simulink model "untitled"  (R2021a)
settings: Solver=VariableStepAuto  StartTime=0.0  StopTime=5  RelTol=1e-3
undefined symbols (not defined in the file or in its folder): sigbuilder_block
libraries: fuzblock x3
(part 2 of 4)

== matlab function untitled/MATLAB Function4 ==
  data: q input; C output; qd input
% Copyright (C) 2022 All rights reserved.
% Authors:     Seonghyeon Jo <cpsc.seonghyeon@gmail.com>
%
% Date:        Jan, 18, 2022
% 
% -------------------------------------------------
% Sawyer Robot 4-DoF
% get a coriolis matrix.
% -------------------------------------------------
% Equation)
%       c(q, dq)
%
% Input)
%       x   : Joint Position
%       dx  : Joint Velocity
% Output)
%       C  : Coriolis Matrix
%
% the following code has been tested on Matlab 2021a
function C = compute_C_4DOF(q,qd)
g=9.81
m1=1;m2=0.7;m3=0.35;
m12=m1+m2;
m23=m2+m3;
m13=m1+m3;
m123=m1+m2+m3;
l1=1;l2=0.7;l3=0.35;
l12=l1*l2;
l23=l2*l3;
l13=l1*l3;
l123=l1*l2*l3;
q1=q(1);
q2=q(2);
q3=q(3);
qd1=qd(1);
qd2=qd(2);
qd3=qd(3);
C1=-m23*l12*sin(q2)*qd2^2-m3*l23*sin(q3)*qd3^2-2*m23*l12*sin(q2)*qd1*qd2-2*m3*l23*sin(q3)*qd2*qd3-2*m3*l23*sin(q3)*qd1*qd3-2*m3*l13*sin(q2+q3)*(qd2+qd3)*(qd1+qd2+qd3);
C2=(m23*l12*sin(q2)+m3*l13*sin(q2+q3))*qd1^2-m3*l23*sin(q3)*qd3^2-2*m3*l23*sin(q3)*qd3*(qd1+qd2);
C3=(m3*l23*sin(q3)+m3*l13*sin(q2+q3))*qd1^2+m3*l23*sin(q3)*qd2^2+2*m3*l23*sin(q3)*qd1*qd2;
C=[C1;C2;C3];
%C = reshape([qd2.*(t2.*(-1.141223459619257e-35)-t3.*5.504493342314691e-37+t241+t252+t255+t266+t276+t284+t304+t310+t322+t336+t346+t353+t360+t367+t375+t384+(t162.*(t234+t236+t237-t3.*t22.*2.206-t8.*t34.*6.053757698066069e-1-t13.*t44.*1.18734317978+t11.*(t37+t41-t3.*t22-t8.*t34.*6.123233995736766e-17).*1.18734317978+t13.*(t37+t41-t3.*t22-t8.*t39.*6.123233995736766e-17).*5.114817050334782e-3))./2.0-(t12.*t215)./2.0-(t129.*t218)./2.0-(t12.*t338)./2.0-(t100.*t286)./2.0-(t7.*t381)./2.0-(t164.*t233)./2.0-(t101.*t317)./2.0-(t121.*t379)./2.0+(t292.*(t20.*(-1.0616375)+t179+t180+t181+t182+t183+t184+t185-t11.*t84.*5.114817050334782e-3+t13.*t84.*1.18734317978))./2.0-(t243.*(t2.*(-2.033158615944436e-19)+t88+t112+t113+t115-t6.*t12.*4.4101e-6-7.623123809914776e-52))./2.0-(t134.*(t5+t9+t80-t6.*t10))./2.0)+qd4.*(t654+t1150+t1160-(t124.*t129)./2.0-(t100.*t164)./2.0-(t101.*t598)./2.0-(t164.*t613)./2.0+(t195.*t692)./2.0+(t162.*(t11.*t53.*5.114817050334782e-3-t13.*t53.*1.18734317978+t11.*t56.*1.18734317978+t13.*t56.*5.114817050334782e-3))./2.0)+qd3.*(t393+t400+t412+t422+t437+t443+t475+t984+t989+t994+t996+(t94.*(t6.*t45.*2.6117415e-2+t8.*t45.*2.799678e-4-t6.*t48.*2.799678e-4+t8.*t48.*2.6117415e-2))./2.0-(t15.*t388)./2.0-(t101.*t398)./2.0-(t129.*t456)./2.0-(t164.*t488)./2.0+(t170.*t492)./2.0+(t195.*t501)./2.0+(t162.*(t6.*t45.*6.053757698066069e-1+t8.*t48.*6.053757698066069e-1+t11.*t150.*5.114817050334782e-3-t13.*t150.*1.18734317978+t11.*t153.*1.18734317978+t13.*t153.*5.114817050334782e-3))./2.0),qd4.*(t654-t1199-t1206+t1582+t1624+t1625+t1982+t1984+t1986+t2555-(t124.*t129)./2.0-(t100.*t164)./2.0-(t101.*t598)./2.0-(t164.*t613)./2.0+(t359.*t1590)./2.0-(t197.*t1910)./2.0-(t1265.*t1911)./2.0+(t1305.*(t1156+t1157+t1158-t1295))./2.0+(t444.*(t1324+t1327+t1331+t1332-t345.*t775-t633.*t783))./2.0)+qd2.*(t2.*(-2.282446919238515e-35)-t3.*1.100898668462938e-36-t1193-t1194-t1195-t1196-t1197+t1270+t120.*(t29+t30)-t12.*t215+t12.*t309+t15.*t321-t12.*t338-t7.*t381+t95.*t366-t242.*t243-t121.*t379+t281.*t1369+t359.*t1305+t177.*t1507+t197.*t1488+t270.*t1662+t303.*t1682+t1155.*t1390+t1265.*t1290+t1251.*t1349+t1227.*t1412-t1254.*t1657+t1252.*t1677+t240.*(t3-t5))+qd1.*(t2.*(-1.141223459619257e-35)-t3.*5.504493342314691e-37+t241+t255+t276+t284+t304+t310+t322+t346+t360+t367+t375+t1234+(t1254.*(t221+t222+t223-t1223-t2.*t727.*2.6811e-2-t3.*t727.*3.0849e-3))./2.0-(t12.*t215)./2.0-(t12.*t338)./2.0-(t100.*t286)./2.0-(t7.*t381)./2.0-(t242.*t243)./2.0-(t121.*t379)./2.0-(t129.*t425)./2.0-(t134.*t530)./2.0-(t101.*t636)./2.0-(t164.*t633)./2.0+(t827.*t1265)./2.0+(t851.*t1251)./2.0+(t1155.*t1190)./2.0+(t1225.*t1227)./2.0+(t1252.*t1666)./2.0)+qd3.*(t393+t400+t412+t422+t437+t443+t475-t848-t852-t885-t909-t910-t973+t1394+t1396+t1783+t1784+t1786+t1788+t1789+t1790+t1791+t1792+t1794+t1796+t1798+t1799+t2069+t2070+t2071+t2072+t2073+t2074+t2075+t2079+t2080-(t15.*t388)./2.0-t242.*t243.*1.874699728327322e-33-(t101.*t398)./2.0-(t129.*t456)./2.0-(t164.*t488)./2.0-(t57.*t1537)./2.0-(t727.*t1544)./2.0),-qd4.*(t1062-t1085+t1086+t1087+t1112+t2022+t2027+t2177+t2197+t2198+t2569+t2570-t124.*t653.*1.874699728327322e-33-(t57.*t1140)./2.0-(t57.*t2185)./2.0-(t197.*t2170)./2.0-(t197.*t2175)./2.0-(t1159.*t1415)./2.0-(t727.*t2024)./2.0-(t1281.*t1474)./2.0-(t1155.*t2180)./2.0-(t1590.*t2028)./2.0)+qd1.*(t393+t400+t412+t422+t437+t443+t475+t984+t994+t2029+t2030-(t15.*t388)./2.0-(t101.*t398)./2.0-(t129.*t456)./2.0-(t164.*t488)./2.0+(t827.*t1782)./2.0+(t1155.*t1803)./2.0+(t197.*(t403+t404+t405+t406-t833-t853))./2.0+(t148.*(t985+t986+t987+t988-t1351-t1352))./2.0)+qd3.*(-t2047-t2060-t2063-t2068+t2088+t2095+t2100+t2112+t2114+t2117+t2137+t2145-t15.*t388.*3.749399456654644e-33-t101.*t398.*3.749399456654644e-33-t129.*t456.*3.749399456654644e-33-t164.*t488.*3.749399456654644e-33+(t57.*t1036)./2.0-t57.*t2042+t177.*t2094+t197.*t2103+t983.*t1467+t1343.*t1378-t727.*t2056-t727.*t2110+t1474.*t1782+t1155.*t2106+t1227.*t2091+(t727.*(t1029+t1030+t1031+t1033+t2043-t2044-t727.*t814))./2.0+t1415.*(t985+t986+t987+t988-t1351-t1352)+(t57.*(t1055+t2061+t2062-t139.*t242.*3.749399456654644e-33-t309.*t444.*3.749399456654644e-33))./2.0+(t727.*(t1039+t1040+t2033-t309.*t806.*3.749399456654644e-33-t727.*t1046-t57.*t2031+t727.*t2032))./2.0)+qd2.*(t393+t400+t412+t422+t437+t443+t475-t848-t852-t885-t909-t910-t973+t1394+t1783+t1786+t1788+t1789+t1790+t1791+t1792+t1794+t1796+t1798+t1799+t2069+t2070+t2071+t2072+t2073+t2074+t2075+t2079+t2080+(t197.*(t1460+t1461+t1462+t1463+t1464-t1872-t1873))./2.0-(t15.*t388)./2.0-t242.*t243.*1.874699728327322e-33-(t101.*t398)./2.0-(t129.*t456)./2.0-(t164.*t488)./2.0-(t57.*t1537)./2.0-(t727.*t1544)./2.0+(t727.*(t1324+t1327+t1331+t1332-t1606-t1607))./2.0),-qd1.*(-t654-t2546-t2548+t2549+t2550+t2552+t2553+(t2307.*t2434)./2.0+(t2539.*t2547)./2.0)-qd3.*(t1062-t1085+t1086+t1087+t1112+t2478+t2558-t2559-t2568+t2569+t2570+t2587+t2648+t2650+t2652-(t1281.*t1474)./2.0-(t444.*t2313)./2.0-(t444.*t2563)./2.0-(t1155.*t2180)./2.0-(t806.*t2566)./2.0-(t2412.*t2434)./2.0-(t2434.*t2435)./2.0)-qd2.*(-t654+t1199+t1206-t1582-t1625-t1982-t1984+t2549+t2550+t2552+t2553-t2555+t2641+t2643+t2644-(t67.*t2441)./2.0-(t444.*t2554)./2.0+(t2472.*t2539)./2.0+(t2434.*t2606)./2.0)-qd4.*(t2618+t2633+t2748+t2753-(t444.*t2543)./2.0-t806.*t2185+t1281.*t1911-(t806.*t2531)./2.0-t1155.*t2626-t2416.*t2539+t2434.*t2636),qd4.*(t654+t1199+t1206-(t45.*(t101.*t565-t124.*t545+t164.*t555))./2.0+(t162.*(t1184+t11.*t53.*1.917749226941314e-35-t13.*t53.*4.451823873129729e-33+t11.*t56.*4.451823873129729e-33+t13.*t56.*1.917749226941314e-35))./2.0-(t162.*(t603.*(t35-t40-t6.*t36+t8.*t39).*5.515+t530.*t609.*5.515+t610.*t647.*5.515+t101.*(t348+t349+t350-t432-t2.*t20.*2.540928714850161e-34+t3.*t22.*4.149651502162508e-18+t6.*t36.*6.776895191416263e-2-t8.*t39.*6.776895191416263e-2).*5.515))./2.0-(t124.*t129)./2.0-(t100.*t164)./2.0-(t101.*t598)./2.0-(t164.*t613)./2.0-(t292.*t714)./2.0+(t427.*t580)./2.0+(t692.*t703)./2.0+(t148.*(t1200+t1201+t1202-t13.*t78.*4.451823873129729e-33-t22.*t640.*5.515))./2.0-(t67.*(t1191+t1192-t124.*t620))./2.0+(t593.*(t20.*(-2.946606165491677e-33)+t584+t585+t587+t588+t589+t590+t591+t592-t11.*t84.*1.917749226941314e-35-t22.*t586.*5.515))./2.0+(t148.*(t1214+t646.*t647.*5.515-t101.*t1211.*5.515-t603.*t1208.*5.515))./2.0+(t444.*(t661+t682+t870+t871-t101.*t681-t164.*t667))./2.0+(t352.*(t101.*t609.*5.515-t603.*t610.*5.515))./2.0)-qd1.*(t2.*(-1.141223459619257e-35)-t3.*5.504493342314691e-37+t241+t252+t255+t266+t276+t284+t304+t310+t322+t336+t346+t353+t360+t367+t375+t384+t1234-(t12.*t215)./2.0-(t129.*t218)./2.0-(t12.*t338)./2.0-(t100.*t286)./2.0-(t7.*t381)./2.0-(t164.*t233)./2.0-(t101.*t317)./2.0-(t242.*t243)./2.0-(t121.*t379)./2.0-(t134.*t426)./2.0+(t162.*(t234+t236+t237-t3.*t22.*2.206-t8.*t39.*6.053757698066069e-1-t13.*t44.*1.18734317978+t11.*t81.*1.18734317978+t13.*t81.*5.114817050334782e-3))./2.0)+qd3.*(t393+t400+t412+t422+t437+t443+t475+t848+t852+t862+t885+t909+t910+t973+(t148.*(t969+t970+t971+t972-t8.*t65.*2.269795582384779e-33-t13.*t139.*4.451823873129729e-33-t520.*(t20-t23).*5.515))./2.0-(t162.*(t121.*(t348+t349+t350+t351-t430-t432+t962-t3.*t22.*2.6e-1).*5.515+t45.*t429.*5.515-t12.*t512.*5.515+t427.*t514.*5.515))./2.0+(t492.*(t917+t918+t920+t921-t6.*t45.*1.049711117200796e-36+t8.*t45.*9.792462161022385e-35-t6.*t48.*9.792462161022385e-35-t8.*t48.*1.049711117200796e-36+t2.*(t20-t23).*1.804608079944675e-33))./2.0-(t94.*(t121.*(t245+t246+t247-t385+t836-t3.*t22.*1.3582e-1).*(3.49e2./2.0e2)-t12.*t483.*(3.49e2./2.0e2)+t45.*t450.*(3.49e2./2.0e2)+t427.*t453.*(3.49e2./2.0e2)))./2.0+(t94.*(t850+t6.*t45.*9.792462161022385e-35+t8.*t45.*1.049711117200796e-36-t6.*t48.*1.049711117200796e-36+t8.*t48.*9.792462161022385e-35))./2.0-t31.*t120.*1.874699728327322e-33-t12.*t309.*1.874699728327322e-33-t15.*t321.*1.874699728327322e-33-(t15.*t388)./2.0-t95.*t366.*1.874699728327322e-33-t124.*t345.*1.874699728327322e-33-(t101.*t398)./2.0-(t129.*t456)./2.0+(t57.*t580)./2.0-(t164.*t488)./2.0-(t22.*t961)./2.0-(t148.*t847)./2.0-(t292.*t711)./2.0-(t111.*t905)./2.0+(t501.*t703)./2.0-(t372.*t976)./2.0+(t162.*(t887+t6.*t45.*2.269795582384779e-33+t8.*t48.*2.269795582384779e-33+t11.*t150.*1.917749226941314e-35-t13.*t150.*4.451823873129729e-33+t11.*t153.*4.451823873129729e-33+t13.*t153.*1.917749226941314e-35))./2.0+(t416.*(t20.*(-9.323350423903855e-34)+t855+t856+t857+t858+t860+t861-t22.*(t2.*(-1.688910400704115e-17)+t417+t418+t419+t493-t6.*t12.*1.6044e-4-5.342894225732868e-34).*(3.49e2./2.0e2)-t6.*t67.*1.049711117200796e-36))./2.0-(t22.*(t661+t682+t426.*(t20.*(-2.881087492837848e-33)+t626+t627+t628+t629+t630-t6.*t65.*7.684130555159526e-1-t8.*t67.*7.684130555159526e-1-t11.*t84.*1.139316919009596e-3+t13.*t84.*8.979785040610579e-2)-t101.*t681-t164.*t667+t425.*(t20.*(-4.271754237092021e-36)+t621+t622+t623+t624+t625+t719-t6.*t65.*1.139316919009596e-3-t8.*t67.*1.139316919009596e-3-t11.*t84.*8.169842925973351e-1)))./2.0+(t829.*(t20.*(-2.946606165491677e-33)+t584+t585+t587+t588+t589+t590+t591+t592-t11.*t84.*1.917749226941314e-35-t22.*(t2.*(-2.449293598294706e-17)+t407+t408+t409+t410+t411+t502-t11.*t15.*9.274373618014111e-4-5.342894225732869e-34).*5.515))./2.0-(t248.*(t121.*t483.*(3.49e2./2.0e2)+t427.*t450.*(3.49e2./2.0e2)))./2.0-(t352.*(t121.*t512.*5.515+t427.*t429.*5.515))./2.0+(t111.*(t906+t907+t908-t8.*t65.*9.792462161022385e-35-t22.*t462.*(3.49e2./2.0e2)))./2.0-(t57.*(t243.*(t892+t893+t894+t2.*t22.*3.3204e-3-t6.*t45.*4.4101e-6+t8.*t45.*2.53e-2-t6.*t48.*2.53e-2-t8.*t48.*4.4101e-6)+t31.*(t889+t890+t891+t2.*t22.*1.4955e-5+t6.*t45.*2.5506e-2-t8.*t45.*4.4101e-6+t6.*t48.*4.4101e-6+t8.*t48.*2.5506e-2)-t95.*(t898-t3.*t22.*3.3204e-3+t6.*t36.*2.53e-2+t8.*t36.*4.4101e-6+t6.*t39.*4.4101e-6-t8.*t39.*2.53e-2)-t121.*(t2.*t20.*(-2.092860147402869e-19)+t3.*t22.*3.4179e-3-t6.*t36.*3.3204e-3+t8.*t36.*1.4955e-5+t6.*t39.*1.4955e-5+t8.*t39.*3.3204e-3)+t15.*(t2.*t20.*(-9.157296440624334e-22)+t3.*t22.*1.4955e-5+t6.*t36.*4.4101e-6+t8.*t36.*2.5506e-2+t6.*t39.*2.5506e-2-t8.*t39.*4.4101e-6)-t12.*(t895+t896+t897+t6.*t45.*1.4955e-5+t8.*t45.*3.3204e-3-t6.*t48.*3.3204e-3+t8.*t48.*1.4955e-5+t2.*(t20-t23).*3.4179e-3)))./2.0),qd2.*(t2.*(-1.141223459619257e-35)-t3.*5.504493342314691e-37+t241+t255+t310+t322+t346+t367+((t57.*t298-t727.*t1666).*(t57.*t1669.*(9.01e2./2.0e2)-t727.*t1672.*(9.01e2./2.0e2)))./2.0+((t57.*t1669-t727.*t1672).*(t57.*t298.*(9.01e2./2.0e2)-t727.*t1666.*(9.01e2./2.0e2)))./2.0-(t12.*t215)./2.0-(t12.*t338)./2.0-(t100.*t286)./2.0-(t7.*t381)./2.0-(t242.*t243)./2.0-(t121.*t379)./2.0-(t129.*t425)./2.0-(t134.*t530)./2.0-(t101.*t636)./2.0-(t164.*t633)./2.0+(t1221.*t1390)./2.0+(t1186.*t1488)./2.0+(t1305.*t1597)./2.0+(t1290.*t1619)./2.0+(t1412.*t1521)./2.0+(t1349.*t1648)./2.0+(t1495.*t1507)./2.0+(t1369.*t1688)./2.0+(t1421.*t1694)./2.0+(t1424.*t1691)./2.0+(t1498.*t1623)./2.0+(t1500.*t1621)./2.0+(t1662.*t1719)./2.0-(t1657.*t1727)./2.0-(t1677.*t1710)./2.0+(t1682.*t1735)./2.0)+qd1.*((t1727.*(t221+t222+t223-t1223-t1728-t1729))./2.0+(t292.*t1186)./2.0-(t281.*t1369)./2.0-(t359.*t1305)./2.0-(t177.*t1507)./2.0-(t197.*t1488)./2.0+(t148.*t1597)./2.0+(t111.*t1688)./2.0+(t372.*t1495)./2.0-(t270.*t1662)./2.0-(t303.*t1682)./2.0+(t275.*t1719)./2.0+(t298.*t1735)./2.0+(t1190.*t1221)./2.0+(t827.*t1619)./2.0+(t851.*t1648)./2.0-(t1155.*t1390)./2.0-(t1265.*t1290)./2.0-(t1251.*t1349)./2.0-(t1227.*t1412)./2.0+(t1225.*t1521)./2.0+(t1254.*t1657)./2.0-(t1252.*t1677)./2.0-(t1666.*t1710)./2.0)+qd3.*(t393+t400+t412+t422+t437+t443+t475+t1394+t1396+t1418+t1459+t1531+t1553+t1914+t1917+t1920+t1927+t1929+t1932+t1935+t1936+t1937+t1938-(t15.*t388)./2.0-(t101.*t398)./2.0-(t129.*t456)./2.0-(t164.*t488)./2.0-(t57.*t1537)./2.0-(t711.*t1488)./2.0-(t878.*t1390)./2.0-(t727.*t1544)./2.0-(t976.*t1507)./2.0+(t1186.*t1400)./2.0+(t1221.*t1478)./2.0-(t1405.*t1412)./2.0+(t1415.*t1597)./2.0+(t1378.*t1648)./2.0-(t1290.*t1742)./2.0-(t1305.*t1738)./2.0+(t1495.*t1557)./2.0+(t1521.*t1564)./2.0+(t1474.*t1619)./2.0-(t1349.*t1746)./2.0-(t1369.*t1749)./2.0+(t1467.*t1688)./2.0-(t1421.*t1764)./2.0+(t1424.*t1769)./2.0-(t1498.*t1774)./2.0+(t1500.*t1779)./2.0-(t1623.*t1771)./2.0+(t1621.*t1776)./2.0-(t1694.*t1763)./2.0+(t1691.*t1768)./2.0+(t1498.*(t1804-t727.*t977))./2.0+(t1186.*(t1460+t1461+t1462+t1463+t1464-t8.*t65.*4.115676486645111e-34-t13.*t139.*8.072210105402954e-34))./2.0)+qd4.*(t654+t1581+t1582+t1624+t1625+t1630+t2007+t2009+t2012+t2013+t2016+t2019-(t124.*t129)./2.0-(t100.*t164)./2.0-(t101.*t598)./2.0-(t164.*t613)./2.0-(t67.*t1603)./2.0+(t444.*t1608)./2.0-(t714.*t1488)./2.0-(t729.*t1639)./2.0+(t1110.*t1390)./2.0+(t1221.*t1575)./2.0+(t1305.*t1610)./2.0-(t1186.*t1910)./2.0+(t1590.*t1597)./2.0-(t1290.*t1974)./2.0+(t1498.*t1871)./2.0-(t1623.*t1806)./2.0-(t1500.*t1967)./2.0+(t1621.*t1855)./2.0-(t1619.*t1911)./2.0),qd3.*(t2087+t2088+t2095+t2096+t2100+t2112+t2113+t2114+t2117+t2118+t2119+t2136+t2137+t2140+t2145+t2148+t2149+t2164+t2384+(t727.*(t2154+t2155+t2156+t2157+t2158-t242.*t1538.*3.749399456654644e-33-t57.*t2163+t321.*(t79-t85).*3.749399456654644e-33))./2.0+t1415.*(t969+t970+t971+t972+t1501-t2085-t2086)-(t727.*(t1832+t1840+t1848+t1849-t2146-t2147+t57.*t1993+t727.*t1990))./2.0-t31.*t120.*7.02899814278107e-66-t12.*t309.*7.02899814278107e-66-t15.*t321.*7.02899814278107e-66-t15.*t388.*3.749399456654644e-33-t95.*t366.*7.02899814278107e-66-t124.*t345.*7.02899814278107e-66-t101.*t398.*3.749399456654644e-33-t129.*t456.*3.749399456654644e-33-t164.*t488.*3.749399456654644e-33-(t57.*t1894)./2.0-t57.*t2042-(t711.*t1400)./2.0-(t878.*t1478)./2.0-(t976.*t1557)./2.0-t727.*t2056-t727.*t2110+t1378.*t1471+t1441.*t1467-(t1405.*t1564)./2.0-(t1378.*t1746)./2.0-(t1415.*t1738)./2.0-(t1467.*t1749)./2.0-(t1474.*t1742)./2.0+t1186.*t2103+t1221.*t2106+t1474.*t1919+t1495.*t2094+t1521.*t2091+t1421.*t2205+t1498.*t2351+t242.*(t80-t323).*7.02899814278107e-66+t1776.*(t1926-t2084)+t1916.*(t1765-t2111)+(t1776.*(t1777+t1778-t1856-t1857))./2.0+(t1771.*(t1772+t1773-t1960-t1961))./2.0+((t1765-t2111).*(t1766+t1767-t1924-t1925))./2.0+((t1760-t1939).*(t1761+t1762-t2138-t2139))./2.0)+qd1.*(t393+t400+t412+t422+t437+t443+t475+t848+t852+t862+t885+t909+t910+t973-t1394-t1396-t1790-t1791-t1792-t1796-t2069-t2071-t2072-t2073-t2074-t2075-t2079-t2080+t2200+t2201+t2202+t2203+(t148.*(t969+t970+t971+t972+t1501-t2085-t2086))./2.0-t31.*t120.*1.874699728327322e-33-(t15.*t388)./2.0-(t101.*t398)./2.0-(t129.*t456)./2.0-(t164.*t488)./2.0+(t57.*t1537)./2.0+(t827.*t1919)./2.0+(t1221.*t1803)./2.0+(t727.*(t1539+t1540+t1541+t1542-t2078+t321.*(t79-t85)))./2.0+(t1186.*(t403+t404+t405+t406-t833-t853))./2.0)+qd2.*(t393+t400+t412+t422+t437+t443+t475+t1914+t1917+t1920+t1927+t1929+t1932+t1935+t1936+t1937+t1938+(t1186.*(t1460+t1461+t1462+t1463+t1464-t1872-t1873))./2.0-(t15.*t388)./2.0-(t101.*t398)./2.0-(t129.*t456)./2.0-(t164.*t488)./2.0+(t1498.*(t1804-t1943))./2.0)-qd4.*(t1062-t1085+t1086+t1087+t1112+t2167+t2172+t2176+t2177+t2181+t2190+t2191+t2192+t2197+t2198+t2602+t2603-t124.*t653.*1.874699728327322e-33-t12.*t1205.*1.874699728327322e-33-t121.*t1198.*1.874699728327322e-33-t444.*t1216.*1.874699728327322e-33-t806.*t1183.*1.874699728327322e-33-(t57.*t2185)./2.0-(t1110.*t1478)./2.0-(t1415.*t1605)./2.0-(t1415.*t1610)./2.0-(t1474.*t1629)./2.0-(t1186.*t2170)./2.0-(t1186.*t2175)./2.0-(t1221.*t2180)./2.0-(t1774.*t1806)./2.0-(t1590.*t2165)./2.0-(t1776.*t2015)./2.0-(t1855.*t2166)./2.0+(t1498.*(t84.*t834+t651.*t734-t646.*t1853-t751.*t1852))./2.0+(t1498.*(t2335-t593.*t806))./2.0),-qd1.*(-t654-t1199-t1206+t1582+t1625+t2549+t2550+t2552+t2553+t2555-t2641-t2642-t2643-t2644-t2645+(t67.*t2441)./2.0+(t444.*t2554)./2.0+(t2307.*t2458)./2.0+(t2547.*t2591)./2.0)-qd4.*(t2618+t2633+t2734+t2742+t2743+t2744+t2745+t2746-(t1110.*t1575)./2.0-(t12.*t2741)./2.0-(t121.*t2738)./2.0-t806.*t2185+t1629.*t1911-t1221.*t2626-(t1911.*t1974)./2.0-t2407.*t2594-t2416.*t2591-(t2404.*t2609)./2.0-(t2407.*t2611)./2.0+t2458.*t2636+t2453.*t2704)-qd3.*(t1062-t1085+t1086+t1087+t1112+t2478-t2559-t2568-t2580-t2582-t2586+t2587-t2588-t2592-t2595+t2602+t2603+t2673+t2674+t2681+t2682+t2683+t2685+t2690+t2691+t2692-(t12.*t2677)./2.0-(t444.*t2313)./2.0-(t121.*t2687)./2.0-(t2412.*t2458)./2.0+(t2302.*t2591)./2.0-(t2299.*t2599)./2.0-(t2363.*t2609)./2.0-(t2416.*t2572)./2.0)-qd2.*(-t654-t2009-t2019+t2549+t2550+t2552+t2553-(t2455.*t2594)./2.0+(t2472.*t2591)./2.0+(t2458.*t2606)./2.0-(t2453.*t2689)./2.0),qd3.*(t2047+t2060+t2063+t2068-(t57.*t1036)./2.0-(t727.*(t1029+t1030+t1031+t1033+t2043-t129.*t766.*3.749399456654644e-33-t727.*t814))./2.0-(t57.*(t1055+t2061+t2062-t139.*t242.*3.749399456654644e-33-t309.*t444.*3.749399456654644e-33))./2.0-(t727.*(t1039+t1040+t2033-t309.*t806.*3.749399456654644e-33-t727.*t1046-t57.*(t1026+t1027+t1043+t1054-t734.*t1004-t806.*t1012)+t727.*(t1023+t1024+t1025+t1041+t1042-t758.*t930)))./2.0)-qd1.*(t393+t400+t412+t422+t437+t443+t475+t984+t989+t994+t996+t2029+t2030-(t15.*t388)./2.0-(t101.*t398)./2.0-(t129.*t456)./2.0-(t164.*t488)./2.0+(t977.*t1155)./2.0+(t827.*(t1333+t1334+t1335+t1336-t11.*t758.*5.114817050334782e-3+t13.*t758.*1.18734317978))./2.0)-qd4.*(t1061+t1062+t1085+t1086+t1087+t1106+t1112+(t444.*(t1029+t1030+t1031+t1033+t57.*t831-t129.*t766.*3.749399456654644e-33-t727.*t814))./2.0-(t444.*(t57.*(t545.*t725+t565.*t722+t555.*t741)+t727.*(t767+t620.*t762-t673.*t766)+t100.*t725.*3.749399456654644e-33+t134.*t722.*3.749399456654644e-33+t129.*t741.*3.749399456654644e-33))./2.0-(t806.*(t818+t820+t1037-t134.*t646.*3.749399456654644e-33-t727.*t831-t57.*(t767+t817-t673.*t766)+t727.*(t815+t816-t766.*t788)))./2.0-t124.*t653.*1.874699728327322e-33-(t148.*t1080)./2.0-(t593.*t711)./2.0+(t714.*t829)./2.0-(t805.*t878)./2.0+(t806.*t1036)./2.0-(t827.*t1115)./2.0-(t977.*t1110)./2.0+(t57.*(t124.*t555+t164.*t545+t124.*(t551+t553-t13.*t53.*4.876002456295764e-2+t11.*t56.*4.876002456295764e-2)-t164.*(-t542+t686+t11.*t53.*8.169842925973351e-1+t13.*t56.*8.169842925973351e-1)-t101.*(t11.*t53.*1.139316919009596e-3-t13.*t53.*8.979785040610579e-2+t11.*t56.*8.979785040610579e-2+t13.*t56.*1.139316919009596e-3)))./2.0-(t827.*(t1120+t1121-t751.*t823.*5.515-t101.*(t825+t826+t828+t1122+t1123-t11.*t758.*9.274373618014111e-4).*5.515))./2.0+(t806.*(t1128+t1132-t101.*t1127-t456.*t788-t164.*t1136+t124.*(t1129+t1130+t1131-t11.*t757.*4.876002456295764e-2-t13.*t757.*2.53401226709415e-4-t13.*t758.*4.876002456295764e-2)))./2.0-(t22.*(t1071+t1073+t164.*t620-t101.*t1067-t164.*t1070))./2.0)-qd2.*(t393+t400+t412+t422+t437+t443+t475+t848+t852+t862+t885+t909+t910+t973+t1418+t1459+t1531+t1553+t2200+t2201+t2202+t2203+(t148.*(t969+t970+t971+t972+t1501-t8.*t65.*2.269795582384779e-33-t13.*t139.*4.451823873129729e-33))./2.0-(t827.*(t1429+t121.*(t962+t964+t965+t966+t967+t1355-t8.*t837.*1.097689519141626e-1-t13.*t883.*2.152934142846781e-1).*5.515-t12.*t876.*5.515+t514.*t806.*5.515))./2.0+(t827.*(t887+t1379+t1380+t1381+t1382-t11.*t758.*1.917749226941314e-35+t13.*t758.*4.451823873129729e-33))./2.0-t31.*t120.*1.874699728327322e-33-t12.*t309.*1.874699728327322e-33-t15.*t321.*1.874699728327322e-33-(t15.*t388)./2.0-t95.*t366.*1.874699728327322e-33-t124.*t345.*1.874699728327322e-33-(t101.*t398)./2.0-(t129.*t456)./2.0-(t164.*t488)./2.0-(t148.*t847)./2.0-(t292.*t711)./2.0-(t111.*t905)./2.0-(t372.*t976)./2.0+(t829.*t1186)./2.0-(t878.*t1190)./2.0+(t977.*t1221)./2.0-(t1225.*t1405)./2.0-(t851.*(t1430-t12.*t978.*(3.49e2./2.0e2)+t453.*t806.*(3.49e2./2.0e2)+t121.*(t836+t914+t915+t916+t1358-t8.*t837.*1.4967e-2).*(3.49e2./2.0e2)))./2.0),-qd1.*(t393+t400+t412+t422+t437+t443+t475+t848+t852+t862+t885+t909+t910+t973+t1418+t1459+t1531+t1553+t1783+t1784+t1786+t1788+t1789-t1790-t1791-t1792+t1794-t1796+t1798+t1799-t31.*t120.*1.874699728327322e-33-(t15.*t388)./2.0-(t101.*t398)./2.0-(t129.*t456)./2.0-(t164.*t488)./2.0-(t292.*t711)./2.0-(t372.*t976)./2.0-(t111.*t1749)./2.0-(t148.*t1738)./2.0-(t878.*t1190)./2.0-(t827.*t1742)./2.0-(t851.*t1746)./2.0-(t1225.*t1405)./2.0)-qd3.*(t2087+t2096+t2113+t2118+t2119+t2136+t2140+t2148+t2149+t2164+t2369+t2389+t2390+(t57.*(t2124+t2125+t2134+t2135-t366.*t758.*3.749399456654644e-33-t242.*t1532.*3.749399456654644e-33-t57.*t2129+t727.*(t2130+t2131+t2132+t2133-t729.*t942+t758.*t948)))./2.0-t31.*t120.*7.02899814278107e-66-t12.*t309.*7.02899814278107e-66-t15.*t321.*7.02899814278107e-66-t95.*t366.*7.02899814278107e-66-t124.*t345.*7.02899814278107e-66-(t57.*t1894)./2.0-(t711.*t1400)./2.0-(t878.*t1478)./2.0-(t976.*t1557)./2.0-(t727.*t1850)./2.0-(t1405.*t1564)./2.0-(t1378.*t1746)./2.0-(t1415.*t1738)./2.0-(t1467.*t1749)./2.0-(t1474.*t1742)./2.0+(t1771.*t1774)./2.0+(t1776.*t1779)./2.0+(t727.*(t2154+t2155+t2156+t2157+t2158+t84.*t321.*3.749399456654644e-33-t242.*t1538.*3.749399456654644e-33-t57.*t2163))./2.0)-qd2.*(t393+t400+t412+t422+t437+t443+t475+t1914+t1917+t1920+t1921+t1922+t1923+t1927+t1929+t1930+t1932+t1933+t1934+t1935+t1936+t1937+t1938+t1941-t31.*t120.*3.749399456654644e-33-t12.*t309.*3.749399456654644e-33-t15.*t321.*3.749399456654644e-33-(t15.*t388)./2.0-t95.*t366.*3.749399456654644e-33-t124.*t345.*3.749399456654644e-33+t242.*t243.*3.749399456654644e-33-(t101.*t398)./2.0+t121.*t379.*3.749399456654644e-33-(t129.*t456)./2.0-(t164.*t488)./2.0+t57.*t1458+t727.*t961-t711.*t1488-t878.*t1390-t976.*t1507-t1405.*t1412-t1290.*t1742-t1305.*t1738+(t1186.*t1909)./2.0-t1349.*t1746-t1369.*t1749+t1424.*t1769+t1500.*t1779-t1623.*t1771+(t1498.*t1942)./2.0-t1694.*t1763)-qd4.*(t1062+t1085+t1086+t1087+t1106+t1112+t1823+t1828+t1908+t1955+t2580-t124.*t653.*1.874699728327322e-33-(t67.*t1036)./2.0-(t711.*t1580)./2.0-(t444.*t1850)./2.0+(t1060.*t1305)./2.0-(t1080.*t1305)./2.0-(t1115.*t1290)./2.0-(t878.*t1575)./2.0-(t878.*t1602)./2.0+(t711.*t1910)./2.0+(t714.*t1909)./2.0-(t1110.*t1514)./2.0-(t729.*t1897)./2.0-(t806.*t1894)./2.0-(t1290.*t1956)./2.0-(t1590.*t1738)./2.0-(t1500.*t1959)./2.0+(t1779.*t1855)./2.0-(t1771.*t1871)./2.0-(t1771.*t1875)./2.0+(t1806.*t1942)./2.0+(t12.*(t2573+t2574+t2575-t100.*t124.*3.749399456654644e-33+t727.*t1603))./2.0+(t121.*(t1921+t1922+t1923+t1930+t1933+t1934+t1941-t124.*t345.*3.749399456654644e-33))./2.0),qd1.*(t2060+t2364+t2368+t2372+t2396-(t727.*(t1039+t1040-t2238+t727.*(t1023+t1025+t1041+t1042-t1053-t1004.*t2233)+t57.*t2279-t727.*t2280-t57.*(t1026+t1027+t1043-t1049-t1050-t960.*t2233)))./2.0+(t57.*(t2281+t2282+t2296-t57.*t2280-t727.*t2279))./2.0+(t416.*t976)./2.0-(t177.*t2094)./2.0+(t57.*t2278)./2.0-(t57.*t2292)./2.0+(t111.*t2285)./2.0+(t993.*t1405)./2.0-(t983.*t1467)./2.0-(t57.*t2566)./2.0+(t878.*t1803)./2.0-(t1343.*t1378)./2.0-(t727.*t2275)./2.0-(t727.*t2313)./2.0+(t851.*t2245)./2.0+(t827.*t2271)./2.0-(t1474.*t1782)./2.0-(t1155.*t2106)./2.0+(t727.*t2557)./2.0-(t727.*t2563)./2.0-(t1227.*t2091)./2.0-(t2028.*t2302)./2.0-(t2103.*t2434)./2.0+(t57.*(-t1038+t2045+t2266+t2268+t2567-t727.*t2263-t57.*(t2264+t2265-t766.*t2248)))./2.0-(t57.*(-t2064+t2281+t2282+t2293+t2296-t727.*(t1026+t1027+t1043-t1049-t1050-t2295)-t57.*(t1023+t1025+t1041+t1042-t1053-t2294)))./2.0+(t2299.*(t403+t404+t405+t406-t833-t853))./2.0+(t2241.*(t140+t141+t142+t143+t144+t146+t147-t205+t2242-t13.*t2233.*2.152934142846781e-1))./2.0)-qd4.*(t2482+t2483+t2489+t2494+t2512+t2513+t2527-t124.*t653.*7.02899814278107e-66+t121.*t1084.*1.874699728327322e-33-(t57.*t2426)./2.0-(t57.*t2509)./2.0-(t1115.*t1474)./2.0+t444.*t2340.*1.874699728327322e-33-(t878.*t2180)./2.0+(t878.*t2199)./2.0+t806.*t2278.*1.874699728327322e-33-(t1110.*t2106)./2.0-(t1474.*t1956)./2.0+(t1911.*t2271)./2.0-(t2103.*t2411)./2.0+(t2241.*t2416)./2.0-(t2299.*t2412)./2.0+(t2302.*t2415)./2.0-(t2299.*t2435)./2.0-(t2343.*t2408)./2.0-(t2351.*t2404)./2.0+(t2363.*t2405)./2.0+(t2362.*t2407)./2.0-(t2302.*t2490)./2.0-(t2363.*t2452)./2.0-(t2343.*t2511)./2.0+(t727.*(t2427+t2429+t806.*t2324))./2.0+(t806.*(t2345+t2347+t2348+t2361-t488.*t766.*3.749399456654644e-33-t100.*t2038.*3.749399456654644e-33+t57.*t2358+t727.*t2360))./2.0-(t121.*(t2088+t2117+t2137-t101.*t398.*3.749399456654644e-33-t129.*t456.*3.749399456654644e-33-t164.*t488.*3.749399456654644e-33+t57.*t2278+t727.*t2340))./2.0-(t444.*(t2318+t2319+t2325+t134.*t2233.*3.749399456654644e-33+t57.*t2324-t442.*t2250.*3.749399456654644e-33-t488.*t2252.*3.749399456654644e-33+t727.*t2327))./2.0)+qd2.*(-t2087-t2096-t2118-t2119-t2136-t2140-t2148-t2149-t2164+t2364+t2368-t2369+t2372-t2384-t2389-t2390+t2396+t120.*(t29+t30).*7.02899814278107e-66+(t2299.*(t1460+t1461+t1462+t1463+t1464-t1872-t1873))./2.0-(t727.*(t2155+t2156+t2157+t2158-t242.*t1538.*3.749399456654644e-33-t321.*t2233.*3.749399456654644e-33-t57.*(t2159+t2160+t2161-t2399-t2400-t1445.*t2233)+t727.*(t2150+t2151+t2153-t2397-t2398-t935.*t2233)))./2.0+t12.*t309.*7.02899814278107e-66+t15.*t321.*7.02899814278107e-66+t95.*t366.*7.02899814278107e-66+t124.*t345.*7.02899814278107e-66-(t57.*t2292)./2.0+(t878.*t1478)./2.0+(t878.*t1514)./2.0+(t976.*t1493)./2.0+(t57.*t2417)./2.0+(t976.*t1557)./2.0+(t57.*t2597)./2.0-(t1378.*t1471)./2.0-(t1441.*t1467)./2.0+(t1405.*t1519)./2.0+(t1405.*t1564)./2.0-(t727.*t2275)./2.0-(t727.*t2313)./2.0+(t1378.*t1746)./2.0-t727.*t2470.*1.874699728327322e-33+(t1467.*t1749)./2.0+(t1474.*t1742)./2.0+(t727.*t2600)./2.0-(t1221.*t2106)./2.0-(t1474.*t1919)./2.0+(t1290.*t2271)./2.0-(t1495.*t2094)./2.0+(t1349.*t2245)./2.0-(t1521.*t2091)./2.0-(t1421.*t2205)./2.0+(t1369.*t2285)./2.0-(t1768.*t1916)./2.0+(t1424.*t2392)./2.0-(t1942.*t2363)./2.0-(t2165.*t2302)./2.0-(t2103.*t2458)./2.0+(t2241.*t2472)./2.0+(t2299.*t2446)./2.0-(t2362.*t2455)./2.0+(t2302.*t2572)./2.0+(t1913.*(t1760-t1939))./2.0+(t2481.*(t1866-t2373))./2.0+(t2601.*(t1962-t2374))./2.0+(t2453.*(t2206-t2365))./2.0+((t1926-t2084).*(t1962-t2374))./2.0)+qd3.*(t57.*(t2345+t2347+t2348+t2361+t57.*(t2346+t751.*t1127-t766.*t1136-t780.*t2038+t762.*t2208+t788.*t2209)+t727.*(t2349+t675.*t734-t762.*t1093-t764.*t2038+t673.*t2209-t751.*t2207)-t488.*t766.*3.749399456654644e-33-t100.*t2038.*3.749399456654644e-33).*(-1.0./2.0)-(t727.*(t120.*t139.*3.749399456654644e-33+t84.*t242.*3.749399456654644e-33-t84.*t388.*3.749399456654644e-33+t139.*t421.*3.749399456654644e-33-t436.*t444.*3.749399456654644e-33-t57.*(t84.*t1008-t139.*t1004-t84.*t2228+t139.*t2222+t444.*t2226)+t727.*(-t84.*t930+t139.*t960+t84.*t2219-t139.*t2212+t444.*t2216)))./2.0+t15.*t134.*7.02899814278107e-66+t95.*t120.*7.02899814278107e-66+t15.*t242.*7.02899814278107e-66-t15.*t388.*7.02899814278107e-66+t100.*t392.*7.02899814278107e-66-t101.*t398.*7.02899814278107e-66+t95.*t421.*7.02899814278107e-66+t121.*t436.*7.02899814278107e-66+t124.*t442.*7.02899814278107e-66-t129.*t456.*7.02899814278107e-66-t164.*t488.*7.02899814278107e-66+t727.*t1105.*1.874699728327322e-33+t57.*t2278.*1.874699728327322e-33+t57.*t2289.*1.874699728327322e-33+(t711.*t2103)./2.0+(t878.*t2106)./2.0-t727.*t2275.*1.874699728327322e-33+(t976.*t2094)./2.0+(t1405.*t2091)./2.0+(t1378.*t2245)./2.0+(t1415.*t2241)./2.0+(t1474.*t2271)./2.0+(t1467.*t2285)./2.0+(t1771.*t2351)./2.0+(t1776.*t2362)./2.0+(t57.*(t120.*t758.*3.749399456654644e-33-t242.*t734.*3.749399456654644e-33+t388.*t734.*3.749399456654644e-33+t421.*t758.*3.749399456654644e-33+t436.*t806.*3.749399456654644e-33+t57.*(t734.*t1008+t758.*t1004-t734.*t2228-t758.*t2222+t806.*t2226)-t727.*(-t734.*t930-t758.*t960+t734.*t2219+t806.*t2216+t2212.*(t750-t754))))./2.0+(t2205.*(t1760-t1939))./2.0+(t2392.*(t1765-t2111))./2.0+(t727.*(t2318+t2319+t2325-t442.*t775.*3.749399456654644e-33-t488.*t783.*3.749399456654644e-33-t134.*(t79-t85).*3.749399456654644e-33+t727.*(t2314+t2315+t2316+t2317+t673.*t2050-t646.*t2207)-t57.*(t84.*t772-t646.*t1127+t783.*t1136-t780.*t2054-t788.*t2050+t775.*t2208)))./2.0),-qd4.*(-t2694-t2695-t2698-t2703+t2712+t2716+t2717+t2729+t121.*t2728+t444.*t2526+t1115.*t1911-t806.*t2509-t878.*t2626+t2416.*t2490-t2407.*t2511+t2299.*t2636+t2363.*t2704-(t2411.*t2697)./2.0)+qd2.*(-t1062-t1085-t1086-t1087-t1112-t1823+t2568+t2587+t2602+t2603+t2673+t2674-t2678+t2681+t2682+t2683+t2685+t2690+t2691+t2692+(t1115.*t1290)./2.0+(t878.*t1602)./2.0-(t12.*t2677)./2.0-(t121.*t2687)./2.0-(t2299.*t2606)./2.0+(t2472.*t2490)./2.0+(t2455.*t2511)./2.0+(t2363.*t2689)./2.0-(t2458.*t2697)./2.0-(t1742.*(t1611-t2004))./2.0-(t2572.*(t1807-t2536))./2.0-(t2736.*(t1866-t2373))./2.0-(t444.*(t2120+t2121+t2123+t2312-t2375-t2376))./2.0-(t2299.*(t1640-t2005-t2006+t2598))./2.0)-qd1.*(t1062+t1085+t1086+t1087+t1112+t1823-t2568-t2569-t2570-t2587-t2648-t2650-t2652+t2678-(t805.*t878)./2.0-(t827.*t1115)./2.0+(t444.*t2313)./2.0+(t444.*t2563)./2.0+(t806.*t2566)./2.0+(t2299.*t2307)./2.0+(t2412.*t2434)./2.0-(t2490.*t2547)./2.0)+qd3.*(-t2482-t2483-t2489-t2494-t2512-t2513-t2527+t2653+t2654+t2655+t2656+t2662+t2663+t2664+t2672),qd4.*((t444.*t1144)./2.0-(t806.*t1140)./2.0+(t806.*t1149)./2.0-(t444.*t2024)./2.0)+qd3.*(t1061+t1062+t1085+t1086+t1087+t1106+t1112+t1823+t1828+t1908+t2022+t2027-(t727.*(t1077+t1145+t1146-t444.*t814+t806.*t831))./2.0-t124.*t653.*1.874699728327322e-33-(t57.*t1140)./2.0-(t148.*t1080)./2.0-(t593.*t711)./2.0-(t805.*t878)./2.0-(t827.*t1115)./2.0-(t977.*t1110)./2.0+(t714.*(t403+t404+t405+t406-t833-t853))./2.0-(t827.*(t1120+t1121-t751.*t823.*5.515-t101.*(t825+t826+t828-t995+t1122+t1123).*5.515))./2.0)-qd1.*(t654+t1150+t1160+t2546+t2548-(t124.*t129)./2.0-(t100.*t164)./2.0-(t101.*t598)./2.0-(t164.*t613)./2.0)-qd2.*(t654+t1199+t1206+t1581+t1630+t1983+t1985+t2642+t2645-(t827.*(t1634+t1635+t1636+t101.*(t964+t965+t966-t1222+t1291-t2.*t20.*2.540928714850161e-34-t3.*t727.*4.149651502162508e-18-t8.*t837.*6.776895191416263e-2).*5.515))./2.0-(t124.*t129)./2.0-(t100.*t164)./2.0-(t101.*t598)./2.0-(t164.*t613)./2.0-(t292.*t714)./2.0-(t67.*t1603)./2.0+(t148.*t1605)./2.0+(t593.*t1186)./2.0-(t729.*t1639)./2.0),qd3.*(t1062+t1085+t1086+t1087+t1106+t1112+t1823+t1828+t1908+t1955+t2167+t2172+t2176+t2181+t2190+t2191+t2192+(t714.*(t1460+t1461+t1462+t1463+t1464-t1872-t1873))./2.0-t124.*t653.*1.874699728327322e-33-t12.*t1205.*1.874699728327322e-33-t121.*t1198.*1.874699728327322e-33-t444.*t1216.*1.874699728327322e-33-t806.*t1183.*1.874699728327322e-33-(t711.*t1580)./2.0-(t1080.*t1305)./2.0-(t1115.*t1290)./2.0-(t878.*t1602)./2.0-(t1110.*t1478)./2.0-(t1110.*t1514)./2.0-(t1415.*t1610)./2.0-(t1290.*t1956)./2.0-(t1500.*t1959)./2.0-(t1774.*t1806)./2.0-(t1771.*t1875)./2.0+(t1806.*(t1804-t1943))./2.0+(t1305.*(t1059-t1898-t1899+t2303))./2.0)-qd1.*(t654+t1199+t1206+t1581+t1630+t1982+t1983+t1984+t1985+t1986-(t124.*t129)./2.0-(t100.*t164)./2.0-(t101.*t598)./2.0-(t164.*t613)./2.0-(t292.*t714)./2.0-(t67.*t1603)./2.0-(t729.*t1639)./2.0+(t1159.*t1305)./2.0-(t827.*t1974)./2.0)-qd2.*(t654+t2007+t2008+t2009+t2010+t2012+t2013+t2016+t2017+t2019+t2020-(t124.*t129)./2.0-(t100.*t164)./2.0-(t101.*t598)./2.0-(t164.*t613)./2.0-t67.*t1603-t714.*t1488-t729.*t1639+t1110.*t1390+t1305.*t1610-t1290.*t1974-t1623.*t1806-t1500.*t1967)+qd4.*((t67.*t1140)./2.0+(t729.*t1144)./2.0+(t444.*t1997)./2.0-(t714.*t1910)./2.0-(t1110.*t1575)./2.0+(t806.*t2003)./2.0-(t1590.*t1610)./2.0+(t1806.*t1871)./2.0+(t1855.*t1967)./2.0-(t1911.*t1974)./2.0-(t12.*(t2619+t2620+t444.*t1603))./2.0-(t121.*(t2008+t2010+t2017+t2020-t67.*t1603-t729.*t1639))./2.0),qd1.*(t1062+t1085+t1086+t1087+t1112+t2459+t2473+t2478+t2558-t124.*t653.*1.874699728327322e-33-(t57.*t2185)./2.0-(t57.*t2531)./2.0+(t57.*t2545)./2.0-(t1281.*t1474)./2.0-(t827.*t1956)./2.0-(t1110.*t1803)./2.0-(t829.*t2411)./2.0+(t727.*t2535)./2.0-(t727.*t2543)./2.0-(t1155.*t2180)./2.0-(t2434.*t2435)./2.0+(t2415.*t2547)./2.0)-qd4.*(t2694+t2695+t2698+t2703-(t121.*t2702)./2.0-(t444.*t2528)./2.0-(t1110.*t2199)./2.0-(t1911.*t1956)./2.0+(t2411.*t2412)./2.0)-qd2.*(-t1062-t1085-t1086-t1087-t1112-t2191-t2192-t2459-t2473-t2478+t2559+t2568+t2582+t2586+t2588+t2592+t2595+t12.*t1205.*1.874699728327322e-33+t121.*t1198.*1.874699728327322e-33+t806.*t1183.*1.874699728327322e-33+(t1110.*t1478)./2.0+(t1110.*t1514)./2.0-t67.*t2578.*1.874699728327322e-33-(t57.*t2623)./2.0+t444.*t2470.*1.874699728327322e-33+(t1290.*t1956)./2.0-(t727.*t2639)./2.0+(t1909.*t2411)./2.0+(t1942.*t2404)./2.0+(t2411.*t2446)./2.0+(t2408.*t2455)./2.0-(t2404.*t2481)./2.0-(t2415.*t2472)./2.0-(t2302.*t2591)./2.0+(t2302.*t2640)./2.0+(t2343.*t2611)./2.0)-qd3.*(-t2482-t2483-t2489-t2494-t2512-t2513-t2527+t2653+t2654+t2655+t2656+t2662+t2663+t2664+t2672-t121.*t1084.*3.749399456654644e-33+t57.*t2426-t444.*t2340.*3.749399456654644e-33+t1110.*t2106-t806.*t2417.*3.749399456654644e-33-t727.*t2528+t1474.*t1956+t2103.*t2411-t2302.*t2415+t2343.*t2408+t2351.*t2404),-qd3.*(t2694+t2695+t2698+t2703-t2712-t2716-t2717-t2729+t806.*t1822.*1.874699728327322e-33+t121.*t2632.*1.874699728327322e-33-(t57.*t2711)./2.0-(t121.*t2728)./2.0+t444.*t2488.*1.874699728327322e-33-(t444.*t2526)./2.0-(t1115.*t1911)./2.0+(t1110.*t2180)./2.0+(t806.*t2509)./2.0+(t727.*t2720)./2.0+(t878.*t2626)./2.0-(t1474.*t2715)./2.0+(t2411.*t2435)./2.0-(t2404.*t2452)./2.0-(t2416.*t2490)./2.0+(t2407.*t2511)./2.0-(t2299.*t2636)./2.0+(t2302.*t2732)./2.0-(t2363.*t2704)./2.0+(t2343.*t2730)./2.0+(t2411.*t2697)./2.0)-qd1.*(t2747-t2748+t2749-t2753+t2754+(t805.*t1110)./2.0-(t444.*t2477)./2.0+(t444.*t2543)./2.0-(t1281.*t1911)./2.0+(t806.*t2531)./2.0-(t827.*t2715)./2.0+(t1155.*t2626)./2.0-(t2307.*t2411)./2.0+(t2416.*t2539)./2.0-(t2434.*t2636)./2.0+(t2547.*t2732)./2.0)-qd4.*((t121.*(t2633+t806.*t1822+t444.*t2488))./2.0+(t444.*t2720)./2.0-(t806.*t2711)./2.0+(t1110.*t2626)./2.0+(t1911.*t2715)./2.0-(t2411.*t2636)./2.0+(t2404.*t2704)./2.0+(t2407.*t2730)./2.0-(t2416.*t2732)./2.0)-qd2.*(-t2734-t2742-t2743-t2744-t2745-t2746+t2747+t2749+t2754+(t1110.*t1575)./2.0+(t1110.*t1602)./2.0+(t12.*t2741)./2.0+(t121.*t2738)./2.0-(t444.*t2477)./2.0-(t1629.*t1911)./2.0+(t1221.*t2626)./2.0+(t1911.*t1974)./2.0-(t1290.*t2715)./2.0+(t2407.*t2594)./2.0+(t2416.*t2591)./2.0-(t2411.*t2606)./2.0+(t2407.*t2611)./2.0-(t2404.*t2689)./2.0-(t2458.*t2636)./2.0+(t2404.*t2736)./2.0-(t2453.*t2704)./2.0+(t2455.*t2730)./2.0+(t2472.*t2732)./2.0)],[4,4]);

== matlab function untitled/MATLAB Function5 ==
  data: q input; G output
% Copyright (C) 2022 All rights reserved.
% Authors:     Seonghyeon Jo <cpsc.seonghyeon@gmail.com>
%
% Date:        Jan, 18, 2022
% 
% -------------------------------------------------
% Sawyer Robot 4-DoF
% get a Gravity vecor
% -------------------------------------------------
% Equation)
%       G(q)
%
% Input)
%       x   : Joint Position
% Output)
%       G  : Gravity Vector
%
% the following code has been tested on Matlab 2021a
function G = compute_G_4DOF(q)
g=9.81
m1=1;m2=0.7;m3=0.35;
m12=m1+m2;
m23=m2+m3;
m13=m1+m3;
m123=m1+m2+m3;
l1=1;l2=0.7;l3=0.35;
l12=l1*l2;
l23=l2*l3;
l13=l1*l3;
l123=l1*l2*l3;
q1=q(1);
q2=q(2);
q3=q(3);
G1=m123*g*l1*cos(q1)+m23*g*l2*cos(q1+q2)+m3*g*l3*cos(q1+q2+q3);
G2=m23*g*l2*cos(q1+q2)+m3*g*l3*cos(q1+q2+q3);
G3=m3*g*l3*cos(q1+q2+q3);
G=[G1;G2;G3];
%G = [0.0;t2.*(-2.754735755355e1)-t3.*1.363342248450017e-1-t13.*(t15+t16).*5.017635526378422e-2+t14.*(t15+t16).*1.16478365936418e1-t7.*t8.*2.746484118e-3-t6.*t10.*2.746484118e-3-t8.*t10.*6.194948142952815-t12.*t13.*1.16478365936418e1-t12.*t14.*5.017635526378422e-2+t6.*(t3-t4).*6.194948142952815;t13.*(t23-t8.*t19.*6.123233995736766e-17).*1.16478365936418e1+t14.*(t23-t8.*t19.*6.123233995736766e-17).*5.017635526378422e-2+t6.*t17.*6.194948142952815-t6.*t19.*2.746484118e-3-t8.*t17.*2.746484118e-3-t8.*t19.*6.194948142952815-t13.*t21.*5.017635526378422e-2+t14.*t21.*1.16478365936418e1;t13.*t27.*(-5.017635526378422e-2)+t14.*t27.*1.16478365936418e1+t13.*(t24-t8.*t19).*1.16478365936418e1+t14.*(t24-t8.*t19).*5.017635526378422e-2];

== matlab function untitled/MATLAB Function6 ==
  data: q input; M output
% Copyright (C) 2022 All rights reserved.
% Authors:     Seonghyeon Jo <cpsc.seonghyeon@gmail.com>
%
% Date:        Jan, 18, 2022
% 
% -------------------------------------------------
% Sawyer Robot 4-DoF
% get a inertia matrix.
% -------------------------------------------------
% Equation)
%       M(q)
%
% Input)
%       x   : Joint Position
% Output)
%       M  : Inertia Matrix
%
% the following code has been tested on Matlab 2021a
function M = compute_M_4DOF(q)
g=9.81
m1=1;m2=0.7;m3=0.35;
m12=m1+m2;
m23=m2+m3;
m13=m1+m3;
m123=m1+m2+m3;
l1=1;l2=0.7;l3=0.35;
l12=l1*l2;
l23=l2*l3;
l13=l1*l3;
l123=l1*l2*l3;
q1=q(1);
q2=q(2);
q3=q(3);
M11=m123*l1^2+m23*l2^2+m3*l3^2+2*m3*l13*cos(q2+q3)+2*m23*l12*cos(q2)+2*m3*l23*cos(q3);
M12=m23*l2^2+m3*l3^2+m3*l13*cos(q2+q3)+m23*l12*cos(q2)+2*m3*l23*cos(q3);
M21=M12;
M13=m3*l3^2+m3*l13*cos(q2+q3)+m3*l23*cos(q3);
M31=M13;
M22=m23*l2^2+m3*l3^2+2*m3*l23*cos(q3);
M23=m3*l3^2+m3*l23*cos(q3);
M32=M23;
M33=m3*l3^2;
M=[M11 M12 M13
    M21 M22 M23
    M31 M32 M33]
%M = reshape([t3.*(-2.282446919238515e-35)+t57+t75+t139+t147+t154-t12.*t85-t60.*t65-t67.*t68-t155.*t160+t100.*t242+t80.*t267+t123.*t247+t109.*t271+t134.*t254+t94.*(t181+t182+t183+t184+t257+t258+t259+t260-t5.*t26.*1.097689519141626e-1-t9.*t55.*9.274373618014111e-4)+(t19.*2.4366e-2+t20.*1.0969e-2).*(t19.*1.296587958e-1+t20.*5.83693397e-2)+(t19.*1.0969e-2-t20.*2.4366e-2).*(t19.*5.83693397e-2-t20.*1.296587958e-1)+2.3659e-2,t3.*(-2.282446919238515e-35)+t57+t75+t139+t147+t154+t242.*(t309+t310+t311+t312-t5.*t23.*1.049711117200796e-36+t7.*t23.*9.792462161022385e-35-t5.*t26.*9.792462161022385e-35-t7.*t26.*1.049711117200796e-36+t2.*(t19-t24).*1.804608079944675e-33)-t12.*t85-t60.*t65-t67.*t68-t155.*t160+(t181+t182+t183+t184+t257+t258+t259+t260-t261-t5.*t26.*1.097689519141626e-1).*(t305+t306+t307+t308+t7.*t23.*2.269795582384779e-33-t5.*t26.*2.269795582384779e-33+t9.*t52.*4.451823873129729e-33-t9.*t55.*1.917749226941314e-35+t13.*t52.*1.917749226941314e-35+t13.*t55.*4.451823873129729e-33+t2.*(t19-t24).*8.271175201380145e-33)+t267.*(t19.*(-1.562776333016795e-33)+t327+t328+t329+t330-t2.*t20.*3.19064476444505e-51+t136.*(t19-t24).*(9.01e2./2.0e2))+t271.*(t19.*(-2.946606165491677e-33)+t339+t340+t341+t342+t343+t344+t345+t346-t13.*t46.*4.451823873129729e-33-t22.*t116.*5.515)+t247.*(t19.*(-9.323350423903855e-34)+t360+t361+t362+t363+t364+t365-t5.*t40.*1.049711117200796e-36-t22.*t128.*(3.49e2./2.0e2))+t254.*(t317+t318+t319-t2.*t19.*3.19064476444505e-51+t2.*t22.*4.528657954898164e-34+t3.*t22.*5.210718333917177e-35-t30.*t136.*(9.01e2./2.0e2))+2.431330457587972e-67,t376+t417+t418+t496+t584-t12.*t85.*3.749399456654644e-33-t60.*t65.*3.749399456654644e-33-t155.*t160.*3.749399456654644e-33-t30.*t546+t247.*t466+t271.*t499-t273.*t524+t554.*t676+t549.*(t238+t239+t240+t299-t406-t407-t408-t413),t448+t678+t685+t271.*t681+t676.*t688,t3.*(-2.282446919238515e-35)+t57+t75+t139+t147+t154+t134.*(t320+t321+t322-t2.*t19.*7.082452307314206e-52+t2.*t22.*1.005251488323677e-34+t3.*t22.*1.156652238383391e-35-t30.*t136)-t12.*t85-t60.*t65-t67.*t68-t155.*t160+t100.*(t313+t314+t315+t316-t5.*t23.*6.015536488256711e-37+t7.*t23.*5.611726166775006e-35-t5.*t26.*5.611726166775006e-35-t7.*t26.*6.015536488256711e-37+t2.*(t19-t24).*1.034159358134484e-33)+t94.*(t301+t302+t303+t304+t7.*t23.*4.115676486645111e-34-t5.*t26.*4.115676486645111e-34+t9.*t52.*8.072210105402954e-34-t9.*t55.*3.477333140419428e-36+t13.*t52.*3.477333140419428e-36+t13.*t55.*8.072210105402954e-34+t2.*(t19-t24).*1.499759782661858e-33)+t109.*(t19.*(-5.342894225732869e-34)+t331+t332+t333+t334+t335+t336+t337+t338-t13.*t46.*8.072210105402954e-34-t22.*t116)+t80.*(t19.*(-3.468981871291444e-34)+t323+t324+t325+t326-t2.*t20.*7.082452307314206e-52+t136.*(t19-t24))+t123.*(t19.*(-5.342894225732868e-34)+t354+t355+t356+t357+t358+t359-t5.*t40.*6.015536488256711e-37-t22.*t128)+2.431330457587972e-67,t3.*(-2.282446919238515e-35)+t57+t75+t139+t147+t154+(-t317-t318-t319+t2.*t19.*3.19064476444505e-51+t30.*t136.*(9.01e2./2.0e2)+t2.*t273.*4.528657954898164e-34+t3.*t273.*5.210718333917177e-35).*(-t320-t321-t322+t2.*t19.*7.082452307314206e-52+t30.*t136+t2.*t273.*1.005251488323677e-34+t3.*t273.*1.156652238383391e-35)+(t30.*t350-t273.*t353).*(t30.*t350.*(9.01e2./2.0e2)-t273.*t353.*(9.01e2./2.0e2))-t12.*t85-t60.*t65-t67.*t68-t155.*t160+t372.*t468+t382.*t461+t414.*t463+t422.*t501+t396.*t559+t410.*t551+(t19.*(-1.562776333016795e-33)+t327+t328+t329+t330-t2.*t20.*3.19064476444505e-51-t136.*t273.*(9.01e2./2.0e2)).*(t19.*(-3.468981871291444e-34)+t323+t324+t325+t326-t2.*t20.*7.082452307314206e-52-t136.*t273)+2.431330457587972e-67,t376+t417+t418+t496+t584-t12.*t85.*3.749399456654644e-33-t60.*t65.*3.749399456654644e-33-t155.*t160.*3.749399456654644e-33-t30.*t546-t273.*t524+t466.*t468+t499.*t501-t463.*t634+t549.*t551+t554.*t559-t461.*(t603-t383.*t420.*5.515),t448+t678+t685+t501.*t681+t559.*t688-t461.*(t695-t430.*t449.*5.515),t376+t417+t418-t22.*(t218+t224+t153.*(t35+t36-t48+t219-t5.*t37-t7.*t40))-t12.*t85.*3.749399456654644e-33-t60.*t65.*3.749399456654644e-33+t30.*t237-t155.*t160.*3.749399456654644e-33+t401.*(t19-t24)+t94.*(t155.*(t181+t182+t183+t184+t387+t388+t389-t5.*t26.*1.097689519141626e-1-t9.*t55.*9.274373618014111e-4+t2.*(t19-t24).*2.6e-1)+t179.*t195)-t30.*(-t55.*t85+t160.*t179+t74.*(t192-t5.*t26))+t100.*(t155.*(t188+t403+t404+t405-t5.*t23.*1.6044e-4-t5.*t26.*1.4967e-2-t7.*t26.*1.6044e-4+t2.*(t19-t24).*1.3582e-1)+t179.*t205)+t123.*(t367+t155.*(t19.*(-8.316576413009676e-18)+t206+t207+t208+t368+t369+t370-t5.*t40.*1.6044e-4))+t109.*(t419+t155.*(t19.*(-1.592040838891559e-17)+t196+t197+t198+t199+t200+t384+t385+t386-t13.*t46.*2.152934142846781e-1)),t376+t417+t418-t12.*t85.*3.749399456654644e-33-t60.*t65.*3.749399456654644e-33-t155.*t160.*3.749399456654644e-33+t30.*t446+t273.*t375-t273.*t401+t372.*t628+t396.*t637-t414.*t632+t410.*t640+t422.*t630+t30.*(t85.*t282-t160.*t383+t74.*(t402-t7.*t275))-t382.*(t602-t383.*t420),t12.*t85.*(-1.405799628556214e-65)-t60.*t65.*1.405799628556214e-65+t69.*t74.*1.405799628556214e-65+t141.*t146.*1.405799628556214e-65+t148.*t153.*1.405799628556214e-65-t155.*t160.*1.405799628556214e-65+t30.*t495.*3.749399456654644e-33-t30.*t546.*3.749399456654644e-33+t30.*t667-t273.*t524.*3.749399456654644e-33+t273.*t583.*3.749399456654644e-33+t273.*t656+t466.*t628+t499.*t630+t549.*t640+t554.*t637+t632.*t634+(t602-t383.*t420).*(t603-t383.*t420.*5.515)-t273.*(-t30.*(-t46.*t531+t193.*t545+t398.*t537)-t273.*(-t46.*t514+t193.*t508+t398.*t522)+t46.*t85.*3.749399456654644e-33+t160.*t193.*3.749399456654644e-33+t74.*t398.*3.749399456654644e-33)+t30.*(t30.*(t282.*t531+t383.*t545-t537.*t601)+t273.*(t282.*t514+t383.*t508-t522.*t601)+t85.*t282.*3.749399456654644e-33-t160.*t383.*3.749399456654644e-33+t74.*t601.*3.749399456654644e-33),t155.*t447.*3.749399456654644e-33+t30.*t699+t193.*t583.*3.749399456654644e-33+t383.*t495.*3.749399456654644e-33+t273.*t703+t630.*t681+t637.*t688+(t602-t383.*t420).*(t695-t430.*t449.*5.515),t437+t448+t94.*(t214.*t229-t148.*(-t182-t183-t184+t261+t431+t432+t433+t2.*t22.*4.149651502162508e-18-t7.*t23.*6.776895191416263e-2+t5.*t26.*6.776895191416263e-2))+t179.*t237+t109.*(t424+t148.*(t20.*(-1.555870108751424e-50)+t196+t197+t199+t425+t426+t427-t3.*t20.*2.540928714850161e-34-t2.*t30.*4.149651502162508e-18-t13.*t46.*2.152934142846781e-1)),t437+t448+t383.*t446+t422.*t672+t396.*(t673+t148.*t452)-t382.*(t675-t430.*t449),t193.*t656+t383.*t667+t499.*t672+t554.*t705+(t675-t430.*t449).*(t603-t383.*t420.*5.515)+t155.*(t417+t418+t496+t584-t60.*t65.*3.749399456654644e-33),t193.*t703+t383.*t699+t672.*t681+t688.*t705+t155.*(t448+t678+t685)+(t675-t430.*t449).*(t695-t430.*t449.*5.515)],[4,4]);
% invM=inv(M)
